simulink model "Cardio_SA_only"  (Simulink 10.2)
settings: Solver=ode1  StartTime=0.0  StopTime=T*16  FixedStep=.00125  RelTol=1e-3  EnableMultiTasking=on
model workspace (MAT data in the model file):
  PulseWidth : num (value not decoded)
PreLoadFcn:
  | %This Model has been adapted from the MATLAB code presented in Hoppensteadt
  | %and Peskin "Modling and Simulation in Medicine and the Life Sciences
  | 
  | %Time parameters
  | T = 0.0125;            % Duration of heartbeat (minutes)
  | Ts = 0.0050;           % Duration of systole   (minutes)
  | Stroke_volume = 70e-3; % L
  | Tmax = 0.0020;         % Time at which flow is maximum (minutes)
  | Qmax= Stroke_volume/(0.5*Ts);    % Maximum flow through aortic valve (liters/minute)
  | dt = .01*T;            % This choice implies 100 timesteps per cardiac cycle
  | 
  | %Systemic arterial and systemic resistance parameters
  | Csa = .003;            % liters/mmHg
  | Rs = 17.86;            % mmHg/(liters/minute)
libraries: simulink x1
settings Model: Creator=bsutton  LastModifiedBy=taylo
settings DataIOCC: LimitDataPoints=on
settings OptimizationCC: ExpressionDepthLimit=2147483647
settings DebuggingCC: SolverPrmCheckMsg=warning  StateNameClashWarn=warning

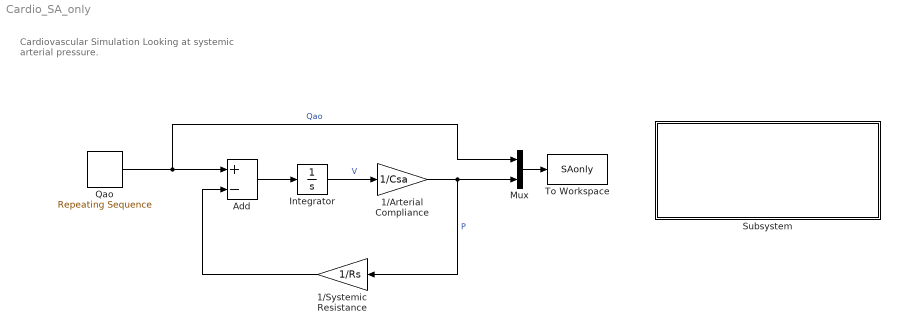
== system Cardio_SA_only ==
  note: Cardiovascular Simulation
      | Looking at systemic arterial pressure.
  1/Arterial Compliance : Gain  Gain=1/Csa
  "1/Systemic Resistance " : Gain  Gain=1/Rs
  Add : Sum  Inputs=+-
  Integrator : Integrator
  Mux : Mux  Inputs=2
  Qao : simulink/Sources/Repeating Sequence  rep_seq_t=[0 Tmax Ts T]  rep_seq_y=[0 Qmax 0 0]
  Subsystem : Subsystem
      mask Display:
      | rgb = imread('Images/Simulink Mask Equations/SA Only.png');
      | image(rgb,'center');
  To Workspace : ToWorkspace  VariableName=SAonly  SaveFormat=Structure With Time  SampleTime=-1
  wires:
  Qao/1 -> Add/1, Mux/1  "Qao"
  "1/Systemic Resistance "/1 -> Add/2
  Mux/1 -> To Workspace/1
  Add/1 -> Integrator/1
  Integrator/1 -> 1/Arterial Compliance/1  "V"
  1/Arterial Compliance/1 -> Mux/2, "1/Systemic Resistance "/1  "P"

== system Cardio_SA_only/Subsystem ==
